simulink model "costant_gain_model"  (R2023b)
settings: Solver=FixedStepAuto  StartTime=0.0  StopTime=10  FixedStep=0.0001  RelTol=1e-3
values from neighbouring files (symbols this model uses):
  Bhip = K_B.K_B.B    [main.m]
  Bknee = K_B.K_B.B    [main.m]
  coef = [2.013+0.1*weight 2+1.344+0.061*weight;0.245*height 0.285*height]    [main.m]
  coef_user = [0.1*weight 0.061*weight; 0.245*height 0.285*height]    [main.m]
  Khip = K_B.K_B.K    [main.m]
  Kknee = K_B.K_B.K    [main.m]
settings Model: Creator=riccardomambrini  LastModifiedBy=riccardomambrini
settings SolverCC: MaxConsecutiveMinStep=100000
settings DebuggingCC: AlgebraicLoopMsg=none

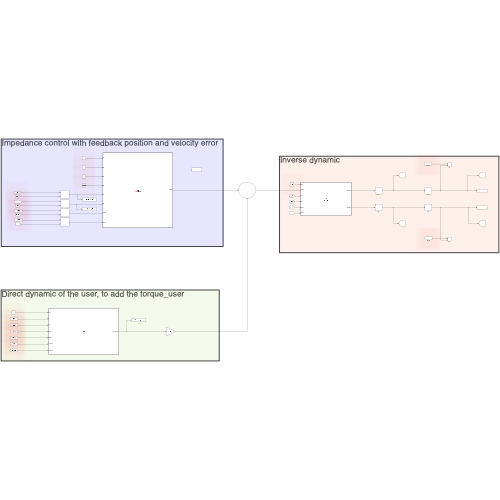
[thumbnail: Simulink's stored preview of the top-level diagram]
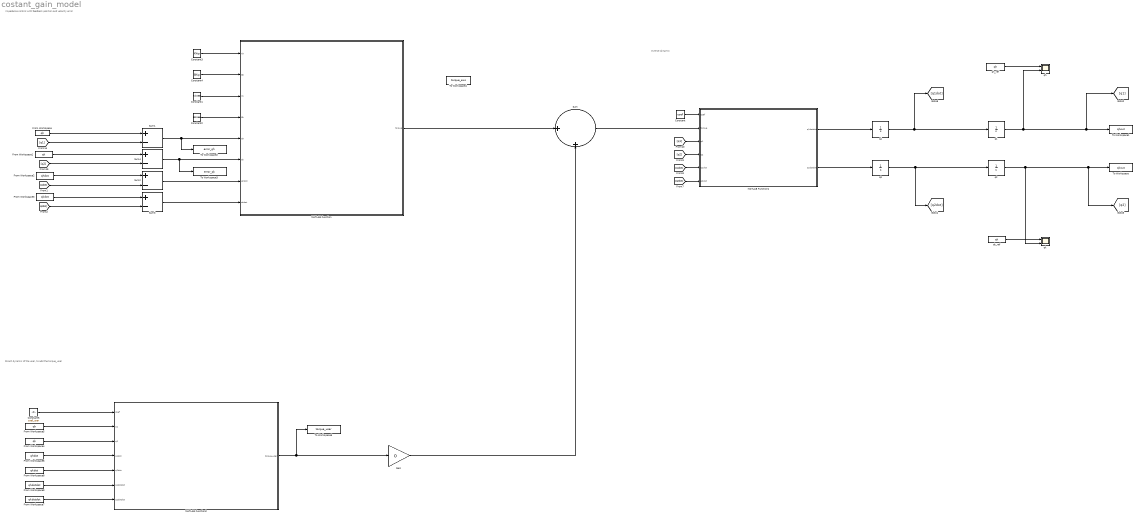
== system costant_gain_model ==
  note: Inverse dynamic
  note: Direct dynamic of the user, to add the torque_user
  note: Impedance control with feedback position and velocity error
  Constant : Constant  Value=coef
  Constant1 : Constant  Value=Kknee
  Constant2 : Constant  Value=Bknee
  Constant3 : Constant  Value=Khip
  Constant4 : Constant  Value=Bhip
  Constant5 : Constant  Value=coef_user
  From Workspace : FromWorkspace  VariableName=qh
  From Workspace1 : FromWorkspace  VariableName=qk
  From Workspace2 : FromWorkspace  VariableName=qhdot
  From Workspace3 : FromWorkspace  VariableName=qkdot
  From Workspace4 : FromWorkspace  VariableName=qk
  From Workspace5 : FromWorkspace  VariableName=qh
  From Workspace6 : FromWorkspace  VariableName=qhdot
  From Workspace7 : FromWorkspace  VariableName=qkdotdot
  From Workspace8 : FromWorkspace  VariableName=qkdot
  From Workspace9 : FromWorkspace  VariableName=qhdotdot
  Gain : Gain  Gain=0
  MATLAB Function : MATLAB Function  TreatAsAtomicUnit=on
  MATLAB Function1 : MATLAB Function  TreatAsAtomicUnit=on
  MATLAB Function2 : MATLAB Function  TreatAsAtomicUnit=on
  Sum : Sum  Inputs=|++
  Sum{1..4} (4 alike) : Sum  Inputs=+-
  To Workspace : ToWorkspace  VariableName=qkout  SampleTime=-1
      settings: MaxDataPoints=100000  Save2DSignal=2-D array (concatenate along first dimension)
  To Workspace1 : ToWorkspace  VariableName=qhout  SampleTime=-1
      settings: MaxDataPoints=100000  Save2DSignal=2-D array (concatenate along first dimension)
  To Workspace2 : ToWorkspace  VariableName=error_qh  SampleTime=-1
      settings: MaxDataPoints=100000  Save2DSignal=2-D array (concatenate along first dimension)
  To Workspace3 : ToWorkspace  VariableName=error_qk  SampleTime=-1
      settings: MaxDataPoints=100000  Save2DSignal=2-D array (concatenate along first dimension)
  To Workspace4 : ToWorkspace  VariableName=torque_exo  SampleTime=-1
      settings: MaxDataPoints=100000  Save2DSignal=2-D array (concatenate along first dimension)
  To Workspace5 : ToWorkspace  VariableName=torque_user  SampleTime=-1
      settings: MaxDataPoints=100000  Save2DSignal=2-D array (concatenate along first dimension)
  q{1..4} (4 alike) : Integrator
  qh : Scope  NumInputPorts=2
  qh_ref : FromWorkspace  VariableName=qh
  qk : Scope  NumInputPorts=2
  qk_ref : FromWorkspace  VariableName=qk
  wires:
  [q1] -> MATLAB Function1/3(q1)
  [q2] -> MATLAB Function1/4(q2)
  [q1dot] -> MATLAB Function1/5(q1dot)
  [q2dot] -> MATLAB Function1/6(q2dot)
  Constant/1 -> MATLAB Function1/1(coef)
  Sum1/1 -> To Workspace2/1, MATLAB Function/5(eh)
  Sum4/1 -> To Workspace3/1, MATLAB Function/6(ek)
  [q2] -> Sum4/2
  From Workspace1/1 -> Sum4/1
  [q1] -> Sum1/2
  From Workspace/1 -> Sum1/1
  Constant3/1 -> MATLAB Function/1(Kh)
  Constant4/1 -> MATLAB Function/2(Bh)
  Constant1/1 -> MATLAB Function/3(Kk)
  Constant2/1 -> MATLAB Function/4(Bk)
  From Workspace5/1 -> MATLAB Function2/2(q1)
  Constant5/1 -> MATLAB Function2/1(coef)
  From Workspace4/1 -> MATLAB Function2/3(q2)
  From Workspace6/1 -> MATLAB Function2/4(q1dot)
  From Workspace8/1 -> MATLAB Function2/5(q2dot)
  From Workspace9/1 -> MATLAB Function2/6(q1dotdot)
  From Workspace7/1 -> MATLAB Function2/7(q2dotdot)
  q2/1 -> qk/2, [q2], To Workspace/1
  MATLAB Function1/2(q2dotdot) -> q3/1
  q3/1 -> [q2dot], q2/1
  MATLAB Function1/1(q1dotdot) -> q4/1
  q4/1 -> [q1dot], q1/1
  q1/1 -> qh/2, [q1], To Workspace1/1
  qh_ref/1 -> qh/1
  qk_ref/1 -> qk/1
  [q1dot] -> Sum2/2
  [q2dot] -> Sum3/2
  From Workspace2/1 -> Sum2/1
  Sum2/1 -> MATLAB Function/7(ehdot)
  From Workspace3/1 -> Sum3/1
  Sum3/1 -> MATLAB Function/8(ekdot)
  MATLAB Function2/1(torque_user) -> To Workspace5/1, Gain/1
  Gain/1 -> Sum/2
  MATLAB Function/1(torque) -> Sum/1
  Sum/1 -> MATLAB Function1/2(torque)

== matlab function costant_gain_model/MATLAB Function1 ==
  data: coef input; q1dotdot output; torque input; q1 input; q2 input; q1dot input; q2dot input; q2dotdot output
function [q1dotdot, q2dotdot]=inverse(coef,torque,q1,q2,q1dot,q2dot)


[q1dotdot, q2dotdot]=inverse_dynamics(coef,torque,q1,q2,q1dot,q2dot);
end

== matlab function costant_gain_model/MATLAB Function ==
  data: Kh input; Bh input; Kk input; Bk input; torque output; eh input; ek input; ehdot input; ekdot input
function torque=impedance(Kh,Bh,Kk,Bk,eh,ek,ehdot,ekdot)

torque=impedance_controller(Kh,Bh,Kk,Bk,eh,ek,ehdot,ekdot);
end

== matlab function costant_gain_model/MATLAB Function2 ==
  data: coef input; torque_user output; q1 input; q2 input; q1dot input; q2dot input; q1dotdot input; q2dotdot input
function torque_user=dynamic_user(coef,q1,q2,q1dot,q2dot,q1dotdot,q2dotdot)

torque_user=dynamic_robot(coef,q1,q2,q1dot,q2dot,q1dotdot,q2dotdot);



end
